simulink model "Cruise_Control_model"  (R2020a)
settings: Solver=VariableStepAuto  StartTime=0.0  StopTime=120  RelTol=1e-3
values from neighbouring files (symbols this model uses):
  b = 50    [controller_design.m]    (also in model_data.sldd = 50.0)
  m = 1000    [controller_design.m]    (also in model_data.sldd = 1000.0)
settings Model: DataDictionary=model_data.sldd  Creator=Viraj  LastModifiedBy=Viraj

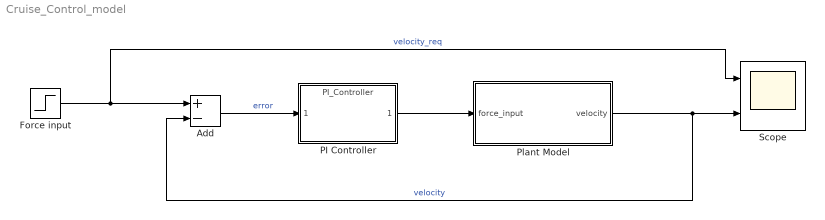
== system Cruise_Control_model ==
  Add : Sum  Inputs=+-
  Force input : Step  After=u  SampleTime=0
  PI Controller : ModelReference  ModelNameDialog=PI_Controller  SimulationMode=Normal  ModelReferenceVersion=1.6
  Plant Model : Subsystem
  Scope : Scope  NumInputPorts=2
  wires:
  Force input/1 -> Add/1, Scope/1  "velocity_req"
  Plant Model/1(velocity) -> Add/2, Scope/2  "velocity"
  Add/1 -> PI Controller/1  "error"
  PI Controller/1 -> Plant Model/1(force_input)

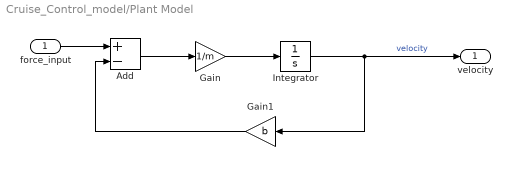
== system Cruise_Control_model/Plant Model ==
  force_input : Inport
  Add : Sum  Inputs=+-
  Gain : Gain  Gain=1/m
  Gain1 : Gain  Gain=b
  Integrator : Integrator
  velocity : Outport
  wires:
  Add/1 -> Gain/1
  Gain/1 -> Integrator/1
  Integrator/1 -> velocity/1, Gain1/1  "velocity"
  Gain1/1 -> Add/2
  force_input/1 -> Add/1
